simulink model "APP"  (R2022b)
settings: Solver=VariableStepAuto  StartTime=0.0  StopTime=15  RelTol=1e-3
settings Model: Creator=MOHAMED  LastModifiedBy=عبدالرحيم
settings SolverCC: AlgebraicLoopSolver=TrustRegion
settings DataIOCC: LoadExternalInput=on
settings DebuggingCC: SFMachineParentedDataDiag=warning  ArithmeticOperatorsInVariantConditions=warning
settings SFSimCC: CustomCodeUndefinedFunction=UseInterfaceOnly

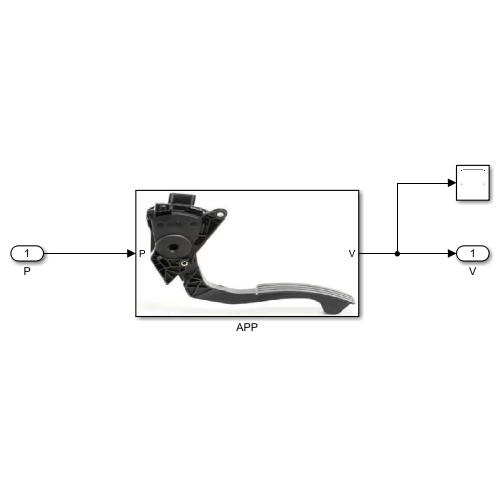
[thumbnail: Simulink's stored preview of the top-level diagram]
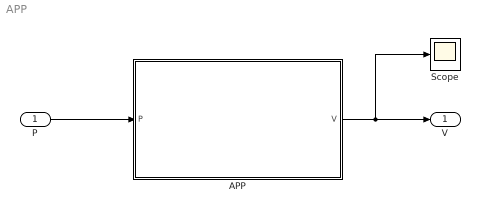
== system APP ==
  P : Inport
  APP : Subsystem
      mask Display: image('WhatsApp Image 2025-03-08 at 23.21.02_ce8e83e1.jpg'); % Use "Edit Image" on toolstrip to change.
  Scope : Scope
  V : Outport
  wires:
  APP/1(V) -> Scope/1, V/1
  P/1 -> APP/1(P)

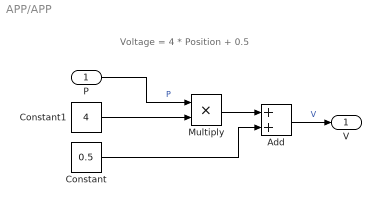
== system APP/APP ==
  note: Voltage = 4 * Position + 0.5
  P : Inport
  Add : Sum
  Constant : Constant  Value=0.5
  Constant1 : Constant  Value=4
  Multiply : Product  Inputs=**
  V : Outport
  wires:
  Constant1/1 -> Multiply/2
  P/1 -> Multiply/1  "P"
  Multiply/1 -> Add/1
  Constant/1 -> Add/2
  Add/1 -> V/1  "V"
